simulink model "Q6"  (R2021b)
settings: Solver=VariableStepAuto  StartTime=0.0  StopTime=30  RelTol=1e-3
settings Model: Creator=DSDLn  LastModifiedBy=DSDLn

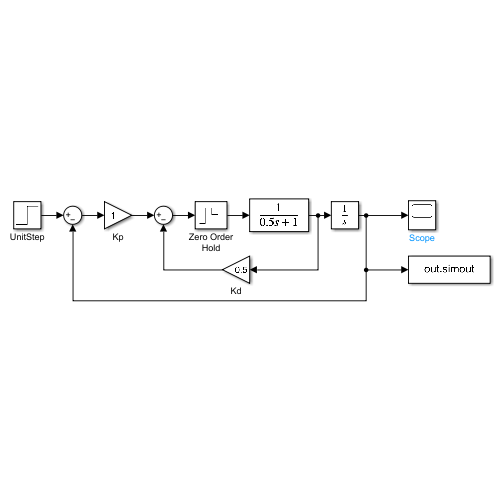
[thumbnail: Simulink's stored preview of the top-level diagram]
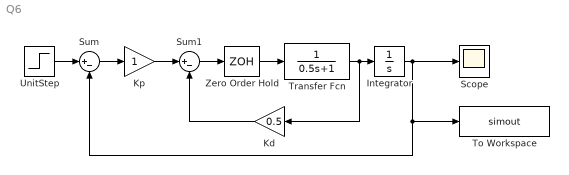
== system Q6 ==
  Integrator : Integrator
  Kd : Gain  Gain=0.5
  Kp : Gain
  Scope : Scope
  Sum : Sum  Inputs=|+-
  Sum1 : Sum  Inputs=|+-
  To Workspace : ToWorkspace  VariableName=simout  SampleTime=-1
  Transfer Fcn : TransferFcn  Denominator=[0.5 1]
  UnitStep : Step  SampleTime=2
  Zero Order Hold : ZeroOrderHold  SampleTime=-1
  wires:
  Sum/1 -> Kp/1
  UnitStep/1 -> Sum/1
  Kp/1 -> Sum1/1
  Sum1/1 -> Zero Order Hold/1
  Zero Order Hold/1 -> Transfer Fcn/1
  Transfer Fcn/1 -> Kd/1, Integrator/1
  Integrator/1 -> To Workspace/1, Sum/2, Scope/1
  Kd/1 -> Sum1/2
